simulink library "math"  (R2016a)
settings: Solver=ode45  StartTime=0.0  StopTime=10.0  RelTol=1e-3
libraries: math x1
settings Model: Creator=jossan  LastModifiedBy=jossan
settings DataIOCC: LimitDataPoints=on
settings DebuggingCC: AllowSymbolicDim=off

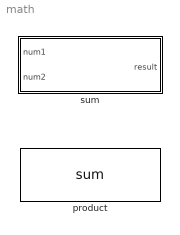
== system math ==
  product : math/sum
  sum : Subsystem

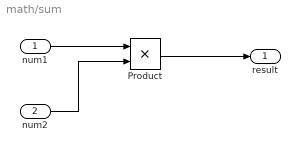
== system math/sum ==
  num1 : Inport  OutDataTypeStr=double
  num2 : Inport  Port=2  OutDataTypeStr=double
  Product : Product
  result : Outport  OutDataTypeStr=double
  wires:
  num1/1 -> Product/1
  num2/1 -> Product/2
  Product/1 -> result/1
